simulink model "commonMetricsValidationSim"  (R2018b)
settings: Solver=FixedStepDiscrete  StartTime=0.0  StopTime=180  FixedStep=0.1  RelTol=1e-3  EnableMultiTasking=on
model workspace (MAT data in the model file):
  ac1_E_ft_0 = 0
  ac1_N_ft_0 = 0
  ac1_a_ftpss_0 = -0.456032315984
  ac1_h_ft_0 = 2989.82506559
  ac1_phi_rad_0 = 0.423268274243
  ac1_psi_rad_0 = 4.56375482858
  ac1_theta_rad_0 = -0.0494964305383
  ac1_v_ftps_0 = 187.614341762
  ac2_E_ft_0 = -29376.3530701
  ac2_N_ft_0 = 43782.7552585
  ac2_a_ftpss_0 = 0
  ac2_h_ft_0 = 1839.62167617
  ac2_phi_rad_0 = 0
  ac2_psi_rad_0 = 2.30640255475
  ac2_theta_rad_0 = 0
  ac2_v_ftps_0 = 229.782865047
libraries: BasicAircraftDynamicsBlock x2, NominalTrajectory x2, CommonMetricsBlock x1
settings Model: Creator=JO20596  LastModifiedBy=BI28030
settings DataIOCC: LimitDataPoints=on  SaveFormat=Array  SignalLoggingSaveFormat=ModelDataLogs
settings OptimizationCC: ExpressionDepthLimit=2147483647  LifeSpan=inf
settings DebuggingCC: UnderspecifiedInitializationDetection=Classic  MergeDetectMultiDrivingBlocksExec=none  SolverPrmCheckMsg=warning  FcnCallInpInsideContextMsg=warning  StateNameClashWarn=warning  SFUnexpectedBacktrackingDiag=warning  SFNoUnconditionalDefaultTransitionDiag=warning  SFExecutionAtInitializationDiag=none
settings HardwareCC: ProdBitPerPointer=32  ProdBitPerSizeT=32  ProdBitPerPtrDiffT=32  ProdLargestAtomicFloat=None  ProdIntDivRoundTo=Undefined  ProdEndianess=Unspecified  ProdWordSize=32  ProdHWDeviceType=32-bit Generic
settings ModelReferenceCC: PropagateSignalLabelsOutOfModel=off
settings SFSimCC: SimUseLocalCustomCode=off
settings RTWCC: RTWUseLocalCustomCode=off
settings CodeAppCC: StateflowObjectComments=on
settings GRTTargetCC: TargetLangStandard=C89/C90 (ANSI)  GeneratePreprocessorConditionals=Disable all  CombineOutputUpdateFcns=off  GRTInterface=on
settings ConfigComp: CovMetricSettings=dw  CovHtmlReporting=on  CovSaveCumulativeToWorkspaceVar=on  CovSaveSingleToWorkspaceVar=on  CovExternalEMLEnable=off

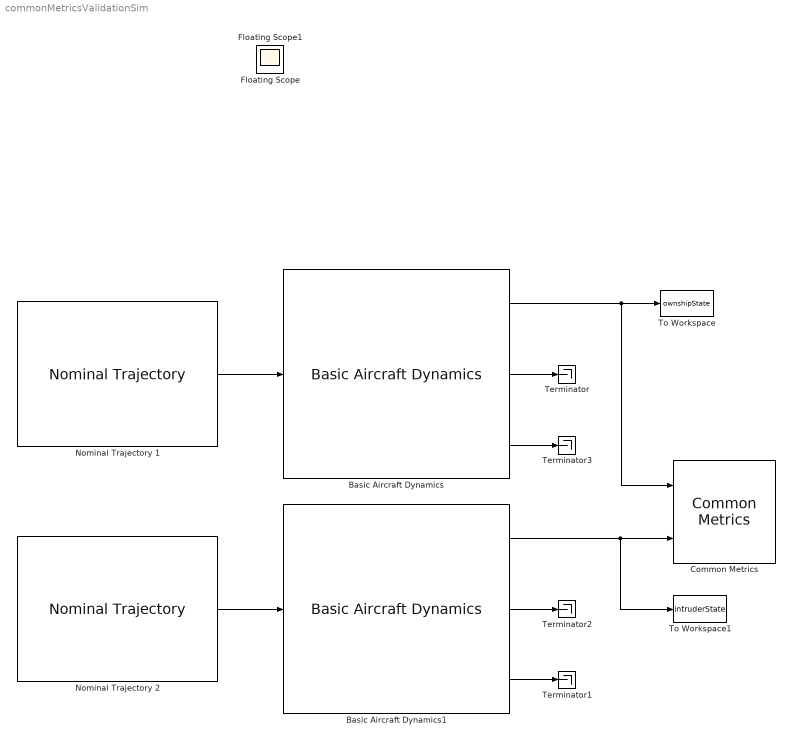
== system commonMetricsValidationSim ==
  Basic Aircraft Dynamics : BasicAircraftDynamicsBlock/Basic Aircraft Dynamics  ts_dynamics=.1  v_ftps_0=ac1dyn_v_ftps  N_ft_0=ac1dyn_N_ft  E_ft_0=ac1dyn_E_ft  h_ft_0=ac1dyn_h_ft  psi_rad_0=ac1dyn_psi_rad  theta_rad_0=ac1dyn_theta_rad  phi_rad_0=ac1dyn_phi_rad  a_ftpss_0=ac1dyn_a_ftpss  v_ftps_max=ac1dyn_con.maxAirspeed_ftps  v_ftps_min=ac1dyn_con.minAirspeed_ftps  dv_ftpss_max=ac1dyn_con.maxAcceleration_ftpss  dv_ftpss_min=ac1dyn_con.minAcceleration_ftpss  dh_ftps_max=ac1dyn_con.maxVerticalRate_ftps  dh_ftps_min=ac1dyn_con.minVerticalRate_ftps  q_radps_max=ac1dyn_con.maxPitchRate_radps  phi_rad_max=ac1dyn_con.maxBankAngle_rad  dphi_radps_max=ac1dyn_con.maxRollRate_radps  r_radps_max=ac1dyn_con.maxYawRate_radps  pNUM=ac1dyn_con.dynamicsNumeratorRollRate  pDEN=ac1dyn_con.dynamicsDenominatorRollRate  hNUM=ac1dyn_con.dynamicsNumeratorVerticalRate  hDEN=ac1dyn_con.dynamicsDenominatorVerticalRate  rNUM=ac1dyn_con.dynamicsNumeratorYawRate  rDEN=ac1dyn_con.dynamicsDenominatorYawRate  lat0_rad=ac2dyn_lat0_rad  lon0_rad=ac2dyn_lon0_rad  alt_ft=ac2dyn_alt0_ft
  Basic Aircraft Dynamics1 : BasicAircraftDynamicsBlock/Basic Aircraft Dynamics  ts_dynamics=.1  v_ftps_0=ac2dyn_v_ftps  N_ft_0=ac2dyn_N_ft  E_ft_0=ac2dyn_E_ft  h_ft_0=ac2dyn_h_ft  psi_rad_0=ac2dyn_psi_rad  theta_rad_0=ac2dyn_theta_rad  phi_rad_0=ac2dyn_phi_rad  a_ftpss_0=ac2dyn_a_ftpss  v_ftps_max=ac2dyn_con.maxAirspeed_ftps  v_ftps_min=ac2dyn_con.minAirspeed_ftps  dv_ftpss_max=ac2dyn_con.maxAcceleration_ftpss  dv_ftpss_min=ac2dyn_con.minAcceleration_ftpss  dh_ftps_max=ac2dyn_con.maxVerticalRate_ftps  dh_ftps_min=ac2dyn_con.minVerticalRate_ftps  q_radps_max=ac2dyn_con.maxPitchRate_radps  phi_rad_max=ac2dyn_con.maxBankAngle_rad  dphi_radps_max=ac2dyn_con.maxRollRate_radps  r_radps_max=ac2dyn_con.maxYawRate_radps  pNUM=ac2dyn_con.dynamicsNumeratorRollRate  pDEN=ac2dyn_con.dynamicsDenominatorRollRate  hNUM=ac2dyn_con.dynamicsNumeratorVerticalRate  hDEN=ac2dyn_con.dynamicsDenominatorVerticalRate  rNUM=ac2dyn_con.dynamicsNumeratorYawRate  rDEN=ac2dyn_con.dynamicsDenominatorYawRate  lat0_rad=ac2dyn_lat0_rad  lon0_rad=ac2dyn_lon0_rad  alt_ft=ac2dyn_alt0_ft
  Common Metrics : CommonMetricsBlock/Common Metrics
  Nominal Trajectory 1 : NominalTrajectory/Nominal Trajectory  eventFilename=event1.mat  ts=.1
  Nominal Trajectory 2 : NominalTrajectory/Nominal Trajectory  eventFilename=event2.mat  ts=.1
  Terminator{,1..3} (4 alike) : Terminator
  To Workspace : ToWorkspace  VariableName=ownshipState  SaveFormat=Timeseries  SampleTime=-1
  To Workspace1 : ToWorkspace  VariableName=intruderState  SaveFormat=Timeseries  SampleTime=-1
  Floating Scope : Scope
  Floating Scope1 : Scope
  wires:
  Basic Aircraft Dynamics/1 -> Common Metrics/1, To Workspace/1
  Nominal Trajectory 1/1 -> Basic Aircraft Dynamics/1
  Basic Aircraft Dynamics/2 -> Terminator/1
  Nominal Trajectory 2/1 -> Basic Aircraft Dynamics1/1
  Basic Aircraft Dynamics1/3 -> Terminator1/1
  Basic Aircraft Dynamics/3 -> Terminator3/1
  Basic Aircraft Dynamics1/2 -> Terminator2/1
  Basic Aircraft Dynamics1/1 -> Common Metrics/2, To Workspace1/1
